simulink model "twoASK"  (R2018a)
settings: Solver=FixedStepAuto  StartTime=0.0  StopTime=40.0  FixedStep=1e-4  RelTol=1e-3
libraries: dsparch4 x1, commrandsrc3 x1
settings Model: Creator=mengmeng  LastModifiedBy=mengmeng

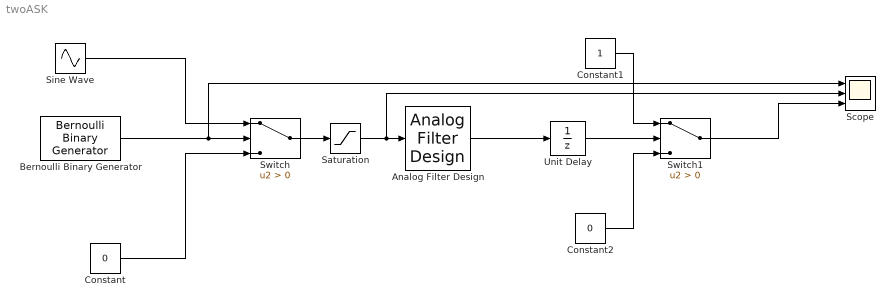
== system twoASK ==
  Analog Filter Design : dsparch4/Analog Filter Design  method=Butterworth  filttype=Lowpass  N=8  Wlo=4*pi  Whi=80  Rp=2  Rs=40
  Bernoulli Binary Generator : commrandsrc3/Bernoulli Binary Generator  ProbabilityOfZero=0.5  SeedSource=Parameter  Seed=61  SampleTime=1  SamplesPerFrame=1  OutputDataType=double  SimulateUsing=Interpreted execution
  Constant : Constant  Value=0
  Constant1 : Constant
  Constant2 : Constant  Value=0
  Saturation : Saturate  UpperLimit=inf  LowerLimit=0
  Scope : Scope  NumInputPorts=3
  Sine Wave : Sin  Frequency=2  SampleTime=0
  Switch : Switch  Criteria=u2 > Threshold
  Switch1 : Switch  Criteria=u2 > Threshold
  Unit Delay : UnitDelay  SampleTime=-1
  wires:
  Sine Wave/1 -> Switch/1
  Bernoulli Binary Generator/1 -> Scope/1, Switch/2
  Constant/1 -> Switch/3
  Switch/1 -> Saturation/1
  Saturation/1 -> Scope/2, Analog Filter Design/1
  Analog Filter Design/1 -> Unit Delay/1
  Unit Delay/1 -> Switch1/2
  Constant1/1 -> Switch1/1
  Constant2/1 -> Switch1/3
  Switch1/1 -> Scope/3
